simulink model "Nonlinear_alg_transform"  (R2016b)
settings: Solver=ode15s  StartTime=0.0  StopTime=300  RelTol=0.01  AbsTol=0.01
settings Model: Creator=Utente  LastModifiedBy=liana
settings SolverCC: MaxOrder=3  MaxConsecutiveMinStep=5  SolverJacobianMethodControl=FullAnalytical  ZeroCrossControl=DisableAll  SolverResetMethod=Robust
settings DataIOCC: SaveState=on
settings OptimizationCC: BlockReduction=off  DefaultParameterBehavior=Inlined  BufferReuse=off

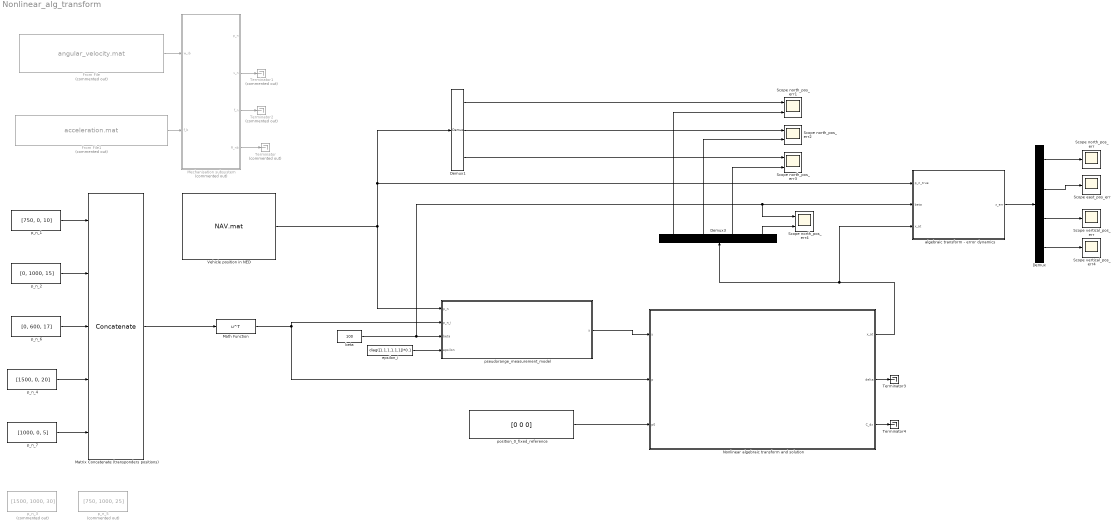
== system Nonlinear_alg_transform ==
  Demux : Demux
  Demux1 : Demux  Outputs=3
  Demux3 : Demux
  From File : FromFile  Commented=on  FileName=angular_velocity.mat  SampleTime=0
  From File1 : FromFile  Commented=on  FileName=acceleration.mat  SampleTime=0
  Math Function : Math  Operator=transpose  SaturateOnIntegerOverflow=on
  Matrix Concatenate (transponders positions) : Concatenate  NumInputs=5  Mode=Multidimensional array  ConcatenateDimension=2
  Mechanisation subsystem : Subsystem  Commented=on
  Nonlinear algebraic transform and solution : Subsystem
  Scope east_pos_err : Scope
  Scope north_pos_err : Scope
  Scope north_pos_err{1..4} (4 alike) : Scope  NumInputPorts=2
  Scope vertical_pos_err : Scope
  Scope vertical_pos_err4 : Scope
  Terminator : Terminator  Commented=on
  Terminator1 : Terminator  Commented=on
  Terminator2 : Terminator  Commented=on
  Terminator3 : Terminator
  Terminator4 : Terminator
  Vehicle position in NED : FromFile  FileName=NAV.mat
  algebraic transform - error dynamics : Subsystem
  beta : Constant  Value=100
  epsilon_i : Constant  Value=diag([1,1,1,1,1,1])*0.1
  p_n_1 : Constant  Value=[750, 0, 10]
  p_n_2 : Constant  Value=[0, 1000, 15]
  p_n_3 : Constant  Commented=on  Value=[1500, 1000, 30]
  p_n_4 : Constant  Value=[1500, 0, 20]
  p_n_5 : Constant  Commented=on  Value=[750, 1000, 25]
  p_n_6 : Constant  Value=[0, 600, 17]
  p_n_7 : Constant  Value=[1000, 0, 5]
  position_0_fixed_reference : Constant  Value=[0 0 0]
  pseudorange_measurement_model : MATLAB Function  TreatAsAtomicUnit=on
  wires:
  pseudorange_measurement_model/1(y) -> Nonlinear algebraic transform and solution/1(y)
  Matrix Concatenate (transponders positions)/1 -> Math Function/1
  p_n_4/1 -> Matrix Concatenate (transponders positions)/4
  p_n_2/1 -> Matrix Concatenate (transponders positions)/2
  p_n_1/1 -> Matrix Concatenate (transponders positions)/1
  Math Function/1 -> pseudorange_measurement_model/2(p_n_i), Nonlinear algebraic transform and solution/2(p)
  p_n_6/1 -> Matrix Concatenate (transponders positions)/3
  beta/1 -> pseudorange_measurement_model/3(beta), Scope north_pos_err4/1, algebraic transform - error dynamics/2(beta)
  From File1/1 -> Mechanisation subsystem/2(f_b)
  From File/1 -> Mechanisation subsystem/1(w_ib)
  Mechanisation subsystem/4(R_nb) -> Terminator/1
  Mechanisation subsystem/2(v_n) -> Terminator1/1
  Mechanisation subsystem/3(f_n) -> Terminator2/1
  Demux/1 -> Scope north_pos_err/1
  Demux/2 -> Scope east_pos_err/1
  Demux/3 -> Scope vertical_pos_err/1
  algebraic transform - error dynamics/1(x_err) -> Demux/1
  Demux1/1 -> Scope north_pos_err1/1
  Demux1/2 -> Scope north_pos_err2/1
  Demux1/3 -> Scope north_pos_err3/1
  Vehicle position in NED/1 -> Demux1/1, algebraic transform - error dynamics/1(p_n_true), pseudorange_measurement_model/1(p_n)
  Nonlinear algebraic transform and solution/1(x_at) -> Demux3/1, algebraic transform - error dynamics/3(x_at)
  epsilon_i/1 -> pseudorange_measurement_model/4(epsilon)
  Demux/4 -> Scope vertical_pos_err4/1
  position_0_fixed_reference/1 -> Nonlinear algebraic transform and solution/3(p0)
  p_n_7/1 -> Matrix Concatenate (transponders positions)/5
  Demux3/1 -> Scope north_pos_err1/2
  Demux3/2 -> Scope north_pos_err2/2
  Demux3/3 -> Scope north_pos_err3/2
  Nonlinear algebraic transform and solution/2(delta) -> Terminator3/1
  Nonlinear algebraic transform and solution/3(C_dx) -> Terminator4/1
  Demux3/4 -> Scope north_pos_err4/2

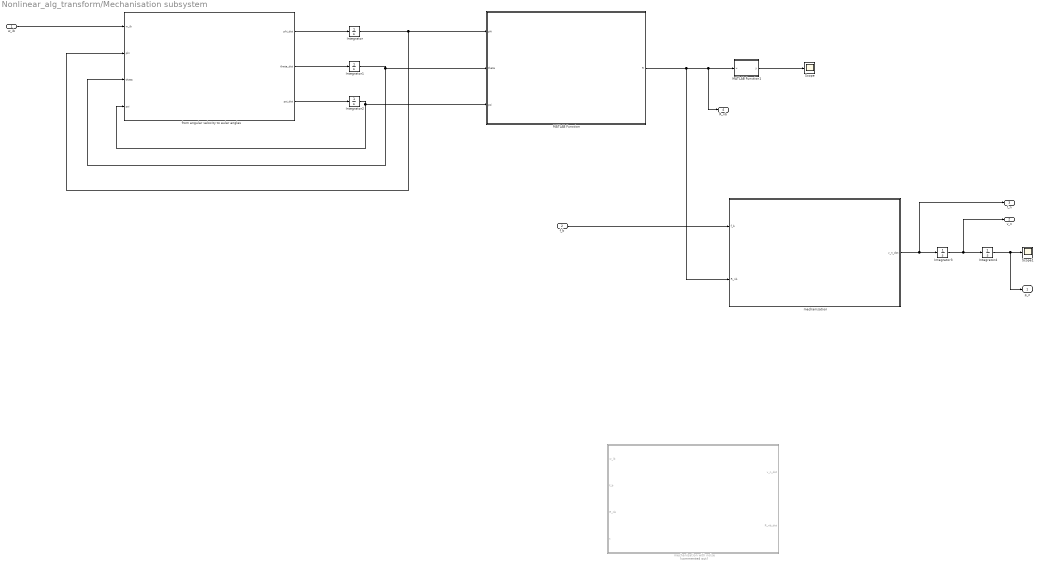
== system Nonlinear_alg_transform/Mechanisation subsystem ==
  w_ib : Inport
  f_b : Inport  Port=2
  Integrator : Integrator  AbsoluteTolerance=0.001
  Integrator1 : Integrator
  Integrator2 : Integrator  AbsoluteTolerance=0.001
  Integrator3 : Integrator
  Integrator4 : Integrator
  MATLAB Function : MATLAB Function  TreatAsAtomicUnit=on
  MATLAB Function1 : MATLAB Function  TreatAsAtomicUnit=on
  Scope : Scope
  Scope1 : Scope
  from angular velocity to euler angles : MATLAB Function  TreatAsAtomicUnit=on
  mechanisation : MATLAB Function  TreatAsAtomicUnit=on
  mechanisation with noise : MATLAB Function  Commented=on  TreatAsAtomicUnit=on
  p_n : Outport
  v_n : Outport  Port=2
  f_n : Outport  Port=3
  R_nb : Outport  Port=4
  wires:
  w_ib/1 -> from angular velocity to euler angles/1(w_ib)
  from angular velocity to euler angles/1(phi_dot) -> Integrator/1
  from angular velocity to euler angles/2(theta_dot) -> Integrator1/1
  from angular velocity to euler angles/3(psi_dot) -> Integrator2/1
  Integrator1/1 -> MATLAB Function/2(theta), from angular velocity to euler angles/3(theta)
  Integrator2/1 -> MATLAB Function/3(psi), from angular velocity to euler angles/4(psi)
  Integrator/1 -> from angular velocity to euler angles/2(phi), MATLAB Function/1(phi)
  MATLAB Function/1(R) -> mechanisation/2(R_nb), R_nb/1, MATLAB Function1/1(u)
  MATLAB Function1/1(y) -> Scope/1
  f_b/1 -> mechanisation/1(f_b)
  Integrator3/1 -> v_n/1, Integrator4/1
  Integrator4/1 -> p_n/1, Scope1/1
  mechanisation/1(v_n_dot) -> f_n/1, Integrator3/1

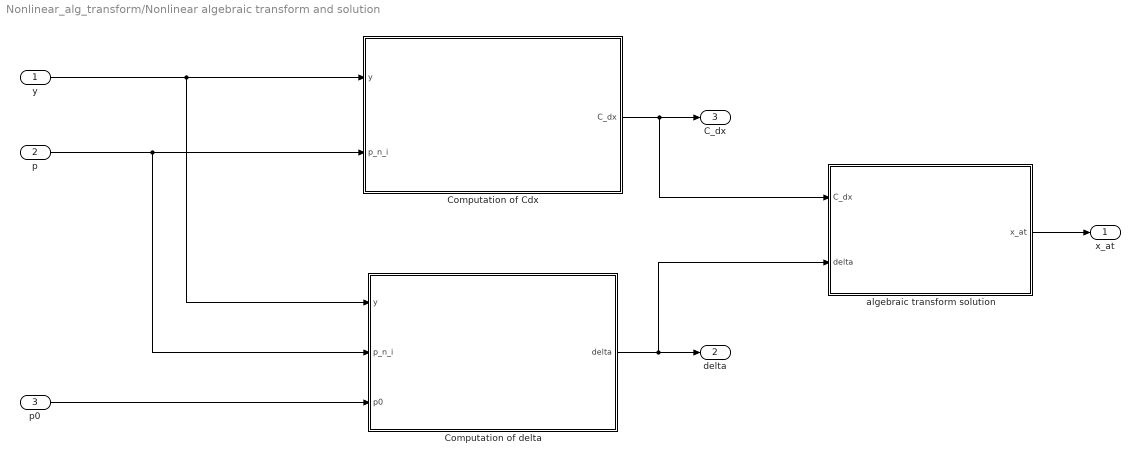
== system Nonlinear_alg_transform/Nonlinear algebraic transform and solution ==
  y : Inport
  p : Inport  Port=2
  p0 : Inport  Port=3
  Computation of Cdx : MATLAB Function  TreatAsAtomicUnit=on
  Computation of delta : MATLAB Function  TreatAsAtomicUnit=on
  algebraic transform solution : MATLAB Function  TreatAsAtomicUnit=on
  x_at : Outport
  delta : Outport  Port=2
  C_dx : Outport  Port=3
  wires:
  y/1 -> Computation of delta/1(y), Computation of Cdx/1(y)
  p/1 -> Computation of delta/2(p_n_i), Computation of Cdx/2(p_n_i)
  p0/1 -> Computation of delta/3(p0)
  Computation of delta/1(delta) -> algebraic transform solution/2(delta), delta/1
  Computation of Cdx/1(C_dx) -> algebraic transform solution/1(C_dx), C_dx/1
  algebraic transform solution/1(x_at) -> x_at/1

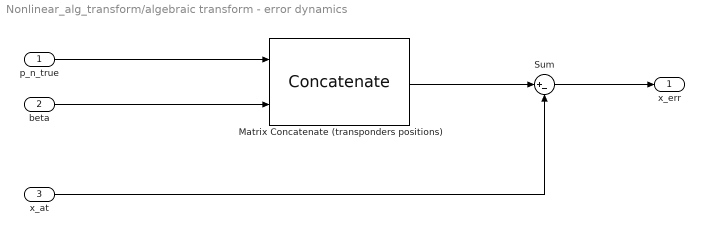
== system Nonlinear_alg_transform/algebraic transform - error dynamics ==
  p_n_true : Inport
  beta : Inport  Port=2
  x_at : Inport  Port=3
  Matrix Concatenate (transponders positions) : Concatenate  Mode=Multidimensional array
  Sum : Sum  Inputs=|+-
  x_err : Outport
  wires:
  p_n_true/1 -> Matrix Concatenate (transponders positions)/1
  beta/1 -> Matrix Concatenate (transponders positions)/2
  x_at/1 -> Sum/2
  Sum/1 -> x_err/1
  Matrix Concatenate (transponders positions)/1 -> Sum/1

== matlab function Nonlinear_alg_transform/Mechanisation subsystem/mechanisation with noise ==
  data: w_ib input; f_b input; v_n_dot output; R_nb_dot output; R_nb input; t input
function [v_n_dot, R_nb_dot] = mechanisation(w_ib, f_b, R_nb, t)



g_n = [0.1 0.1 9.81]';

% w_ib = size(3,1);

if t == 0
    v_n_dot = zeros(3,1);
    R_nb_dot = eye(3);
    R_nb = eye(3);
end

Skew = skew(w_ib);


%p_dot = v_n;

v_n_dot = R_nb * f_b + g_n;

R_nb_dot = R_nb * Skew;

== matlab function Nonlinear_alg_transform/Nonlinear algebraic transform and solution/Computation of Cdx ==
  data: y input; p_n_i input; C_dx output
function C_dx  = C_dx_func(y,p_n_i)

    % y vector 
    % p matrix has row vectors
    %            (x,y,z) cols 
    %            m-rows are transponders number
    % all variables are in navigation frame oh yeah! baby ;)
    
    [row,col] = size(p_n_i);
    [row_,col_] = size(y);
    
    % m-measure vector
    p_m = p_n_i(row,:); % measure of m-th transponder
    y_m = y(row_);  % m-th pseudorange measure

    m = row; % m is transpoders number
    
    
    p_ = zeros(m-1,3); %row vector, 3 stands for x,y,z
    y_ = zeros(m-1,1);
    
    for i = 1 : 1 : m-1
    
        p_(i,:) = p_m - p_n_i(i,:);
        y_(i) = y(i) - y_m;
        
    end
    
    C_dx = [p_, y_];

end

== matlab function Nonlinear_alg_transform/Nonlinear algebraic transform and solution/Computation of delta ==
  data: y input; delta output; p_n_i input; p0 input
function delta   = delta_func(y, p_n_i, p0)

    % y vector 
    % p matrix has row vectors
    %            (x,y,z) cols 
    %            m-rows are the numbers of the transponders
    % all variables are in navigation frame oh yeah! baby ;)
    % z is a col vector of scalars
    
    % we must choose p0 (a block)
    
    [row,col] = size(p_n_i);
    %[row_,col_] = size(y);
    
    p_los = zeros(row,col);
    z = zeros(row,1);   % dim = m x 1
    
    %defining los vector
    for i = 1:1:row
       p_los(i,:) = p_n_i(i,:) - p0';       % dim = m x 3
    end
    
%     p_n_true = p_los;
    
    % p_los = p_los';
    
    for i = 1:1:row
        z(i)= ((y(i)^2) - norm(p_los(i,:))^2); % dim = m x 1
    end
    
%     z = z';
%     
%     delta = zeros(row-1,1);
%     z_m = z(end);
%     
%     for i = 1:1:row-1
%         delta(i) =  (z(i) - z_m); %amm fenito
%     end

    delta = zeros(row-1,1); %dim = (m-1) x 1
    z_m = z(row,1);
    
    for i=1:1:(row-1)
        delta(i,1) = z(i,1) - z_m;
    end

end

== matlab function Nonlinear_alg_transform/pseudorange_measurement_model ==
  data: p_n input; y output; p_n_i input; beta input; epsilon input
function y = pseudorange_mea_model(p_n, p_n_i, beta, epsilon)

  %  row-vector

  y = zeros(size(p_n_i,1),1);

  for i = 1:1:size(p_n_i,1)

      rho = norm(p_n - (p_n_i(i,:))');  % eq. 7
      
      y(i) = rho + beta + epsilon(i); % eq. 8 

  end
      
end

== matlab function Nonlinear_alg_transform/Mechanisation subsystem/from angular velocity to euler angles ==
  data: w_ib input; phi input; theta input; psi input; phi_dot output; theta_dot output; psi_dot output
function [phi_dot, theta_dot, psi_dot] = w2doteuler(w_ib, phi, theta, psi)


D = zeros(3,3);
D(1,1) = 1;
D(1,2) = sin(phi)*tan(theta);
D(1,3) = cos(phi)*tan(theta);

D(2,2) = cos(phi);
D(2,3) = -sin(phi);

D(3,2) = sin(phi)/cos(theta);
D(3,3) = cos(phi)/cos(theta); 


% D = [ 1    sin(phi)*tan(theta)     cos(phi)*tan(theta);
%       0        cos(phi)                - sin(phi);
%       0    sin(phi)/cos(theta)     cos(phi)/cos(theta)]; 

phi_dot = D(1,:) * w_ib;
theta_dot = D(2,:) * w_ib;
psi_dot = D(3,:) * w_ib;

end

== matlab function Nonlinear_alg_transform/Mechanisation subsystem/MATLAB Function ==
  data: phi input; R output; theta input; psi input
function R = eul2R(phi, theta, psi)

angles = [phi theta psi];

R = eul2rotm(angles,'ZYX');

end

== matlab function Nonlinear_alg_transform/Mechanisation subsystem/MATLAB Function1 ==
  data: u input; y output
function y = fcn(u)

y = norm(u);

== matlab function Nonlinear_alg_transform/Mechanisation subsystem/mechanisation ==
  data: f_b input; v_n_dot output; R_nb input
function v_n_dot  = mechanisation(f_b, R_nb)

g_n = [0.1 0.1 9.81]';

v_n_dot = R_nb * f_b + g_n;

end

== matlab function Nonlinear_alg_transform/Nonlinear algebraic transform and solution/algebraic transform solution ==
  data: C_dx input; x_at output; delta input
function x_at = solAT(C_dx, delta)

% this solution is described in the Appendix
% that is correct only for m >= 5

pC_dx = pinv(C_dx);

x_at = pC_dx * (delta / 2);

end
